simulink model "lotkavolterra_simu"  (R2021a)
settings: Solver=ode45  StartTime=0.0  StopTime=10  MaxStep=5e-3  RelTol=1e-3  EnableMultiTasking=on
settings Model: Creator=nicolas  LastModifiedBy=fernando
settings SolverCC: AlgebraicLoopSolver=TrustRegion
settings DataIOCC: SaveFormat=Array  ReturnWorkspaceOutputs=off
settings OptimizationCC: LifeSpan=inf
settings DebuggingCC: AllowSymbolicDim=off  SFUnexpectedBacktrackingDiag=warning  SFNoUnconditionalDefaultTransitionDiag=warning  SFExecutionAtInitializationDiag=none  SFMachineParentedDataDiag=warning  ArithmeticOperatorsInVariantConditions=warning
settings HardwareCC: ProdBitPerPointer=32  ProdBitPerSizeT=32  ProdBitPerPtrDiffT=32  ProdLargestAtomicFloat=None  ProdIntDivRoundTo=Undefined  ProdEndianess=Unspecified  ProdWordSize=32  ProdHWDeviceType=32-bit Generic
settings ModelReferenceCC: PropagateSignalLabelsOutOfModel=off
settings SFSimCC: SimUseLocalCustomCode=off  CustomCodeUndefinedFunction=UseInterfaceOnly
settings RTWCC: RTWUseLocalCustomCode=off
settings CodeAppCC: StateflowObjectComments=on
settings GRTTargetCC: TargetLangStandard=C89/C90 (ANSI)
settings ConfigComp: CovMetricSettings=dw  CovSaveCumulativeToWorkspaceVar=on  CovSaveSingleToWorkspaceVar=on  CovExternalEMLEnable=off

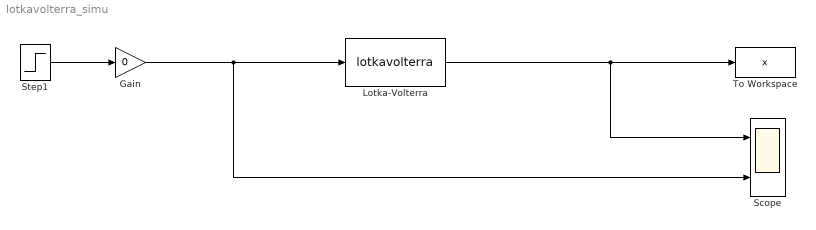
== system lotkavolterra_simu ==
  Gain : Gain  Gain=0
  Lotka-Volterra : S-Function  FunctionName=lotkavolterra  Parameters=x0  SFunctionDeploymentMode=off  EnableBusSupport=off
  Scope : Scope  NumInputPorts=2
  Step1 : Step  Time=2  After=5  SampleTime=0
  To Workspace : ToWorkspace  VariableName=x  SampleTime=-1
  wires:
  Step1/1 -> Gain/1
  Lotka-Volterra/1 -> Scope/1, To Workspace/1
  Gain/1 -> Lotka-Volterra/1, Scope/2
